simulink model "sistem_3"  (R2026a)
settings: Solver=VariableStepAuto
settings Model: Creator=ASUS  LastModifiedBy=ASUS

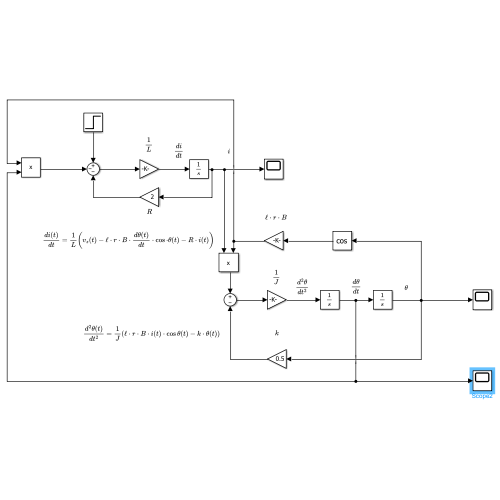
[thumbnail: Simulink's stored preview of the top-level diagram]
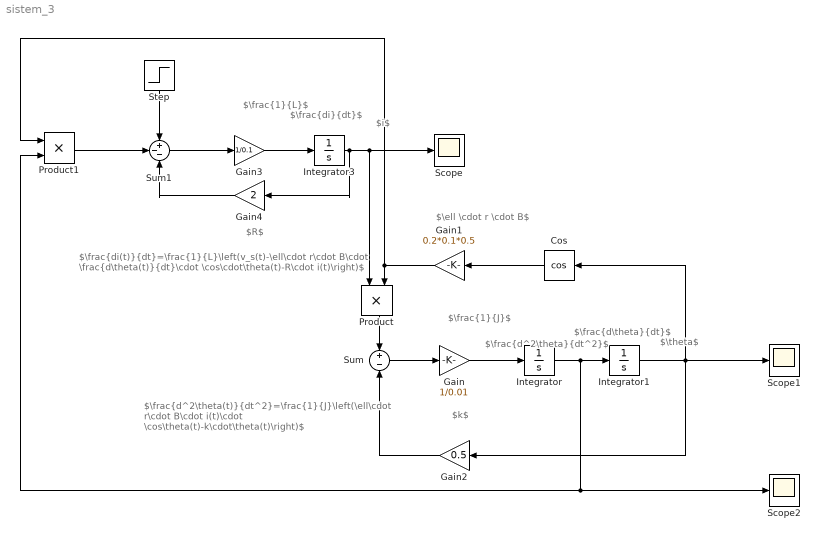
== system sistem_3 ==
  note: $\frac{di(t)}{dt}=\frac{1}{L}\left(v_s(t)-\ell\cdot r\cdot B\cdot \frac{d\theta(t)}{dt}\cdot \cos\cdot\theta(t)-R\cdot i(t)\right)$
  note: $\frac{1}{J}$
  note: $\ell \cdot r \cdot B$
  note: $\theta$
  note: $\frac{d\theta}{dt}$
  note: $\frac{d^2\theta}{dt^2}$
  note: $\frac{di}{dt}$
  note: $i$
  note: $k$
  note: $\frac{d^2\theta(t)}{dt^2}=\frac{1}{J}\left(\ell\cdot r\cdot B\cdot i(t)\cdot \cos\theta(t)-k\cdot\theta(t)\right)$
  note: $\frac{1}{L}$
  note: $R$
  Cos : Trigonometry  Operator=cos
  Gain : Gain  Gain=1/0.01
  Gain1 : Gain  Gain=0.2*0.1*0.5
  Gain2 : Gain  Gain=0.5
  Gain3 : Gain  Gain=1/0.1
  Gain4 : Gain  Gain=2
  Integrator : Integrator
  Integrator1 : Integrator  InitialCondition=0.1
  Integrator3 : Integrator
  Product : Product
  Product1 : Product
  Scope : Scope
      settings: ActiveDisplayYMinimum=-1.5120071928423862  ActiveDisplayYMaximum=7.1804798255839657
  Scope1 : Scope
      settings: ActiveDisplayYMinimum=-0.14151990373054046  ActiveDisplayYMaximum=0.2745845605246936
  Scope2 : Scope
      settings: ActiveDisplayYMinimum=-1.0110640465386977  ActiveDisplayYMaximum=1.0120263226113118  DataLoggingVariableName=ScopeData2
  Step : Step  FinalValue=12  SampleTime=0
  Sum : Sum  Inputs=+-
  Sum1 : Sum  Inputs=+--
  wires:
  Integrator/1 -> Product1/2, Scope2/1, Integrator1/1
  Sum/1 -> Gain/1
  Gain/1 -> Integrator/1
  Integrator1/1 -> Gain2/1, Scope1/1, Cos/1
  Cos/1 -> Gain1/1
  Product/1 -> Sum/1
  Integrator3/1 -> Gain4/1, Scope/1, Product/1
  Gain1/1 -> Product1/1, Product/2
  Gain2/1 -> Sum/2
  Gain3/1 -> Integrator3/1
  Sum1/1 -> Gain3/1
  Step/1 -> Sum1/1
  Product1/1 -> Sum1/2
  Gain4/1 -> Sum1/3
